simulink model "hr_PID"  (R2024b)
settings: Solver=VariableStepAuto  StartTime=0.0  StopTime=T  RelTol=1e-3
values from neighbouring files (symbols this model uses):
  a = 1    [bifurcation_diagram.m]    (also in equilibria.m; flow.m; flow_analysis.m; linear_analysis.m)
  A = hr_jacobian(x_eq, a, b, d, r, s)    [params.m]
  b = 3    [bifurcation_diagram.m]    (also in equilibria.m; flow.m; flow_analysis.m; linear_analysis.m = linspace(0, 10, 100))
  B = [1; 0; 0]    [params.m]
  c = 1    [bifurcation_diagram.m]    (also in equilibria.m; flow.m; flow_analysis.m; linear_analysis.m)
  C = [1, 0, 0]    [params.m]
  d = 5    [bifurcation_diagram.m]    (also in equilibria.m; flow.m; flow_analysis.m; linear_analysis.m)
  D = 0    [params.m]
  d_filter = 100    [params.m]
  I = linspace(1.2, 3.5, 1000)    [bifurcation_diagram.m]    (also in equilibria.m = 1.309; flow.m = 1.3059; linear_analysis.m = 2; params.m = 1.28)
  Kd = 2.67    [params.m]
  Ki = 49.48    [params.m]
  Kp = 108.97    [params.m]
  r = 0.003    [bifurcation_diagram.m]    (also in equilibria.m; flow.m; flow_analysis.m; linear_analysis.m = 0.001)
  s = 4    [bifurcation_diagram.m]    (also in equilibria.m; flow.m; flow_analysis.m; linear_analysis.m)
  uncertainty = 0    [params.m]    (also in plot_sim_reg.m; plot_sim_reg_disturbance.m; plot_sim_reg_uncertainties.m = 1; plot_sim_track.m)
  x_0 = [0.1; 0.1; 0.1]    [bifurcation_diagram.m]    (also in flow.m = x_0_generic; params.m; plot_sim_track.m = hr_equilibria(a,b,c,d,s,x_r,I); plot_sim_track_disturbance.m = hr_equilibria(a,b,c,d,s,x_r,I))
  x_eq = current_eq(1, j)    [linear_analysis.m]    (also in params.m = eq(1,1); plot_sim_track.m = eq(1,1); plot_sim_track_disturbance.m = eq(1,1); plot_sim_track_uncertainties.m = eq(1,1))
  x_r = -8/5    (= -1.6)    [bifurcation_diagram.m]    (also in equilibria.m; flow.m; flow_analysis.m; linear_analysis.m)
libraries: slpidlib x2
settings Model: Creator=vincip  LastModifiedBy=vincip

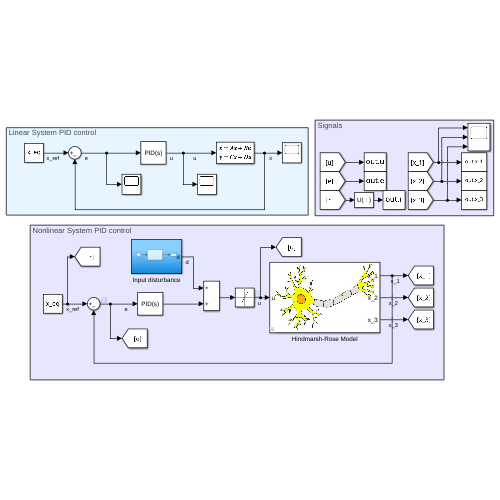
[thumbnail: Simulink's stored preview of the top-level diagram]
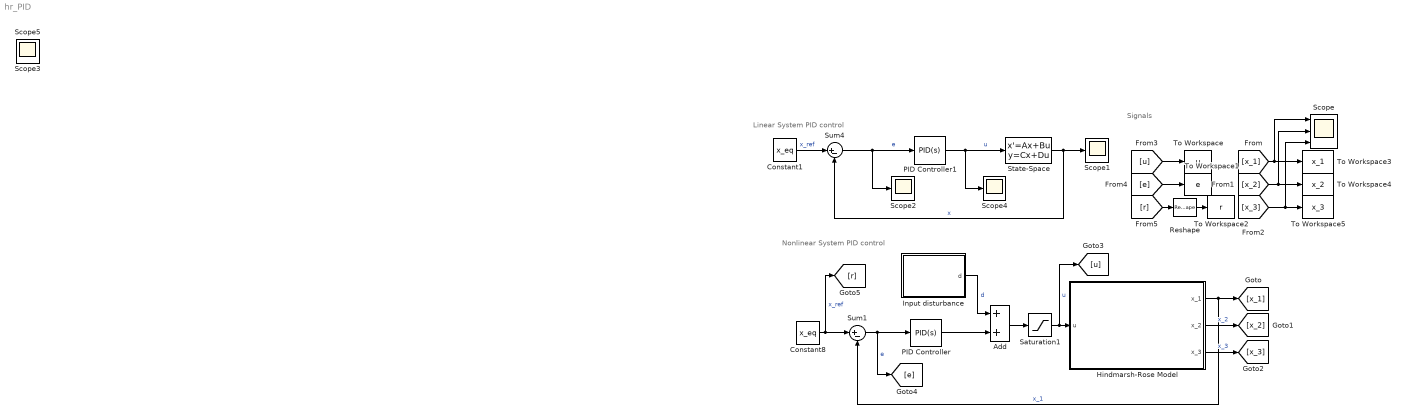
== system hr_PID ==
  note: Signals
  note: Linear System PID control
  note: Nonlinear System PID control
  Add : Sum
  Constant1 : Constant  Value=x_eq
  Constant8 : Constant  Value=x_eq
  Hindmarsh-Rose Model : Subsystem  mask{a=a, b=b, c=c, d=d, r=r, s=s, x_r=x_r, I=I, x_0=x_0, uncertainty=uncertainty}
      mask DialogControl DescTextVar Prompt: Hindmarsh-Rose Neuronal Model with an external input u
      mask Display:
      | image('figures/neuron.jpg');
      | port_label('input', 1, 'u');
      | port_label('output', 1, 'x_1');
      | port_label('output', 2, 'x_2');
      | port_label('output', 3, 'x_3');
  Input disturbance : Subsystem
  PID Controller : slpidlib/PID Controller  Controller=PID  Form=Parallel  TimeDomain=Continuous-time  UseExternalTs=off  SampleTime=-1  IntegratorMethod=Forward Euler  FilterMethod=Forward Euler  ControllerParametersSource=internal  P=Kp  I=Ki  UseKiTs=off  D=Kd  UseExternalDerivativeSource=off  N=d_filter  UseFilter=on  TunerSelectOption=Transfer Function Based (PID Tuner App)  InitialConditionSource=internal  InitialConditionForIntegrator=0  InitialConditionForFilter=0  DifferentiatorICPrevScaledInput=0  ExternalReset=none  TrackingMode=off  Kt=1  LimitOutput=off  SatLimitsSource=internal  UpperSaturationLimit=inf  LowerSaturationLimit=-inf  LinearizeAsGain=on  AntiWindupMode=none  Kb=1  LimitIntegrator=off  UpperIntegratorSaturationLimit=inf  LowerIntegratorSaturationLimit=-inf  POutMin=[]  POutMax=[]  IOutMin=[]  IOutMax=[]  DOutMin=[]  DOutMax=[]  NOutMin=[]  NOutMax=[]  SumOutMin=[]  SumOutMax=[]  SaturationOutMin=[]  SaturationOutMax=[]  PParamMin=[]  PParamMax=[]  IParamMin=[]  IParamMax=[]  DParamMin=[]  DParamMax=[]  NParamMin=[]  NParamMax=[]  KbParamMin=[]  KbParamMax=[]  KtParamMin=[]  KtParamMax=[]  KbOutMin=[]  KbOutMax=[]  KtOutMin=[]  KtOutMax=[]  IntegratorOutMin=[]  IntegratorOutMax=[]  FilterOutMin=[]  FilterOutMax=[]  SumI1OutMin=[]  SumI1OutMax=[]  SumI2OutMin=[]  SumI2OutMax=[]  SumI3OutMin=[]  SumI3OutMax=[]  SumI4OutMin=[]  SumI4OutMax=[]  SumDOutMin=[]  SumDOutMax=[]  DifferentiatorOutMin=[]  DifferentiatorOutMax=[]  FilterDiffOutCoefMin=[]  FilterDiffOutCoefMax=[]  ReciprocalOutMin=[]  ReciprocalOutMax=[]  SumDenOutMin=[]  SumDenOutMax=[]  SumNumOutMin=[]  SumNumOutMax=[]  DivideOutMin=[]  DivideOutMax=[]  UdiffTsProdOutMin=[]  UdiffTsProdOutMax=[]  NTsProdOutMin=[]  NTsProdOutMax=[]  UintegralTsProdOutMin=[]  UintegralTsProdOutMax=[]  UngainTsProdOutMin=[]  UngainTsProdOutMax=[]  ClampingZeroOutDataTypeStr=Inherit: Inherit via back propagation  ClampingZeroOutMin=[]  ClampingZeroOutMax=[]  FilterDenConstantOutDataTypeStr=Inherit: Inherit via back propagation  FilterDenConstantOutMin=[]  FilterDenConstantOutMax=[]  PCopyOutDataTypeStr=Inherit: Inherit via back propagation  PCopyOutMin=[]  PCopyOutMax=[]  NCopyOutDataTypeStr=Inherit: Inherit via back propagation  NCopyOutMin=[]  NCopyOutMax=[]  IntegratorContinuousStateAttributes=''  IntegratorStateMustResolveToSignalObject=off  IntegratorRTWStateStorageClass=Auto  FilterContinuousStateAttributes=''  FilterStateMustResolveToSignalObject=off  FilterRTWStateStorageClass=Auto  ParallelPVariant=InternalParameters  IdealPVariant=Disabled  IVariant=InternalParameters  DVariant=InternalParameters  IntegratorVariant=Continuous  SatVariant=Disabled  AWVariant=Passthrough  PCopyVariant=Disabled  TRVariant=Disabled  FdbkBlocksVariant=Forward  IdealPFdbkVariant=Disabled  SatFdbkVariant=Disabled  DerivativeFilterVariant=ContFilter  NVariant=InternalParameters  NCopyVariant=Disabled  FilterICVariant=InternalICsFilter  IntegratorICVariant=InternalICs  ExternalResetVariant=Disabled  TRSumVariant=Passthrough  SumFdbkVariant=Disabled  SumVariant=Sum_PID  TsampFilterVariant=InternalTs  TsampNgainVariant=Passthrough  TsampIntegralVariant=Disabled_SignalSpec  ExternalSaturationOutDataTypeStr=Inherit: Same as second input  DerivativeSourceVariant=ErrorSignal  PreIntVariant=InternalPreInt
  PID Controller1 : slpidlib/PID Controller  Controller=PID  Form=Parallel  TimeDomain=Continuous-time  UseExternalTs=off  SampleTime=-1  IntegratorMethod=Forward Euler  FilterMethod=Forward Euler  ControllerParametersSource=internal  P=Kp  I=Ki  UseKiTs=off  D=Kd  UseExternalDerivativeSource=off  N=d_filter  UseFilter=on  TunerSelectOption=Transfer Function Based (PID Tuner App)  InitialConditionSource=internal  InitialConditionForIntegrator=0  InitialConditionForFilter=0  DifferentiatorICPrevScaledInput=0  ExternalReset=none  TrackingMode=off  Kt=1  LimitOutput=off  SatLimitsSource=internal  UpperSaturationLimit=inf  LowerSaturationLimit=-inf  LinearizeAsGain=on  AntiWindupMode=none  Kb=1  LimitIntegrator=off  UpperIntegratorSaturationLimit=inf  LowerIntegratorSaturationLimit=-inf  POutMin=[]  POutMax=[]  IOutMin=[]  IOutMax=[]  DOutMin=[]  DOutMax=[]  NOutMin=[]  NOutMax=[]  SumOutMin=[]  SumOutMax=[]  SaturationOutMin=[]  SaturationOutMax=[]  PParamMin=[]  PParamMax=[]  IParamMin=[]  IParamMax=[]  DParamMin=[]  DParamMax=[]  NParamMin=[]  NParamMax=[]  KbParamMin=[]  KbParamMax=[]  KtParamMin=[]  KtParamMax=[]  KbOutMin=[]  KbOutMax=[]  KtOutMin=[]  KtOutMax=[]  IntegratorOutMin=[]  IntegratorOutMax=[]  FilterOutMin=[]  FilterOutMax=[]  SumI1OutMin=[]  SumI1OutMax=[]  SumI2OutMin=[]  SumI2OutMax=[]  SumI3OutMin=[]  SumI3OutMax=[]  SumI4OutMin=[]  SumI4OutMax=[]  SumDOutMin=[]  SumDOutMax=[]  DifferentiatorOutMin=[]  DifferentiatorOutMax=[]  FilterDiffOutCoefMin=[]  FilterDiffOutCoefMax=[]  ReciprocalOutMin=[]  ReciprocalOutMax=[]  SumDenOutMin=[]  SumDenOutMax=[]  SumNumOutMin=[]  SumNumOutMax=[]  DivideOutMin=[]  DivideOutMax=[]  UdiffTsProdOutMin=[]  UdiffTsProdOutMax=[]  NTsProdOutMin=[]  NTsProdOutMax=[]  UintegralTsProdOutMin=[]  UintegralTsProdOutMax=[]  UngainTsProdOutMin=[]  UngainTsProdOutMax=[]  ClampingZeroOutDataTypeStr=Inherit: Inherit via back propagation  ClampingZeroOutMin=[]  ClampingZeroOutMax=[]  FilterDenConstantOutDataTypeStr=Inherit: Inherit via back propagation  FilterDenConstantOutMin=[]  FilterDenConstantOutMax=[]  PCopyOutDataTypeStr=Inherit: Inherit via back propagation  PCopyOutMin=[]  PCopyOutMax=[]  NCopyOutDataTypeStr=Inherit: Inherit via back propagation  NCopyOutMin=[]  NCopyOutMax=[]  IntegratorContinuousStateAttributes=''  IntegratorStateMustResolveToSignalObject=off  IntegratorRTWStateStorageClass=Auto  FilterContinuousStateAttributes=''  FilterStateMustResolveToSignalObject=off  FilterRTWStateStorageClass=Auto  ParallelPVariant=InternalParameters  IdealPVariant=Disabled  IVariant=InternalParameters  DVariant=InternalParameters  IntegratorVariant=Continuous  SatVariant=Disabled  AWVariant=Passthrough  PCopyVariant=Disabled  TRVariant=Disabled  FdbkBlocksVariant=Forward  IdealPFdbkVariant=Disabled  SatFdbkVariant=Disabled  DerivativeFilterVariant=ContFilter  NVariant=InternalParameters  NCopyVariant=Disabled  FilterICVariant=InternalICsFilter  IntegratorICVariant=InternalICs  ExternalResetVariant=Disabled  TRSumVariant=Passthrough  SumFdbkVariant=Disabled  SumVariant=Sum_PID  TsampFilterVariant=InternalTs  TsampNgainVariant=Passthrough  TsampIntegralVariant=Disabled_SignalSpec  ExternalSaturationOutDataTypeStr=Inherit: Same as second input  DerivativeSourceVariant=ErrorSignal  PreIntVariant=InternalPreInt
  Reshape : Reshape
  Saturation1 : Saturate  UpperLimit=10  LowerLimit=-10  LinearizeAsGain=off  ZeroCross=off
  Scope : Scope  NumInputPorts=3
  Scope{1..5} (5 alike) : Scope
  State-Space : StateSpace  A=A  B=B  C=C  D=D  InitialCondition=x_0
  Sum1 : Sum  Inputs=|+-
  Sum4 : Sum  Inputs=|+-
  To Workspace : ToWorkspace  VariableName=u  SaveFormat=Timeseries  SampleTime=-1
  To Workspace1 : ToWorkspace  VariableName=e  SaveFormat=Timeseries  SampleTime=-1
  To Workspace2 : ToWorkspace  VariableName=r  SaveFormat=Timeseries  SampleTime=-1
  To Workspace3 : ToWorkspace  VariableName=x_1  SaveFormat=Timeseries  SampleTime=-1
  To Workspace4 : ToWorkspace  VariableName=x_2  SaveFormat=Timeseries  SampleTime=-1
  To Workspace5 : ToWorkspace  VariableName=x_3  SaveFormat=Timeseries  SampleTime=-1
  wires:
  Constant8/1 -> [r], Sum1/1  "x_ref"
  PID Controller/1 -> Add/2
  Add/1 -> Saturation1/1
  Sum1/1 -> [e], PID Controller/1  "e"
  PID Controller1/1 -> State-Space/1, Scope4/1  "u"
  Sum4/1 -> Scope2/1, PID Controller1/1  "e"
  Constant1/1 -> Sum4/1  "x_ref"
  State-Space/1 -> Scope1/1, Sum4/2  "x"
  Input disturbance/1(d) -> Add/1  "d"
  Saturation1/1 -> [u], Hindmarsh-Rose Model/1(u)  "u"
  Hindmarsh-Rose Model/2(x_2) -> [x_2]  "x_2"
  Hindmarsh-Rose Model/3(x_3) -> [x_3]  "x_3"
  Hindmarsh-Rose Model/1(x_1) -> Sum1/2, [x_1]  "x_1"
  [x_1] -> To Workspace3/1, Scope/1
  [x_2] -> To Workspace4/1, Scope/2
  [x_3] -> To Workspace5/1, Scope/3
  [u] -> To Workspace/1
  [e] -> To Workspace1/1
  [r] -> Reshape/1
  Reshape/1 -> To Workspace2/1

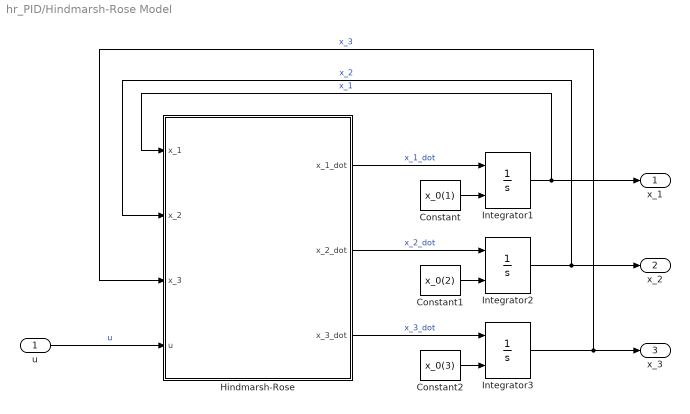
== system hr_PID/Hindmarsh-Rose Model ==
  u : Inport
  Constant : Constant  Value=x_0(1)
  Constant1 : Constant  Value=x_0(2)
  Constant2 : Constant  Value=x_0(3)
  Hindmarsh-Rose : MATLAB Function  TreatAsAtomicUnit=on
  Integrator1 : Integrator  InitialConditionSource=external  InitialCondition=x_0
  Integrator2 : Integrator  InitialConditionSource=external  InitialCondition=x_0
  Integrator3 : Integrator  InitialConditionSource=external  InitialCondition=x_0
  x_1 : Outport
  x_2 : Outport  Port=2
  x_3 : Outport  Port=3
  wires:
  Hindmarsh-Rose/2(x_2_dot) -> Integrator2/1  "x_2_dot"
  Integrator1/1 -> Hindmarsh-Rose/1(x_1), x_1/1  "x_1"
  Hindmarsh-Rose/3(x_3_dot) -> Integrator3/1  "x_3_dot"
  Integrator3/1 -> x_3/1, Hindmarsh-Rose/3(x_3)  "x_3"
  u/1 -> Hindmarsh-Rose/4(u)  "u"
  Hindmarsh-Rose/1(x_1_dot) -> Integrator1/1  "x_1_dot"
  Integrator2/1 -> Hindmarsh-Rose/2(x_2), x_2/1  "x_2"
  Constant/1 -> Integrator1/2
  Constant1/1 -> Integrator2/2
  Constant2/1 -> Integrator3/2

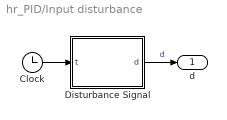
== system hr_PID/Input disturbance ==
  Clock : Clock
  Disturbance Signal : MATLAB Function  TreatAsAtomicUnit=on
  d : Outport
  wires:
  Clock/1 -> Disturbance Signal/1(t)
  Disturbance Signal/1(d) -> d/1  "d"

== matlab function hr_PID/Hindmarsh-Rose Model/Hindmarsh-Rose ==
  data: x_1 input; x_2 input; x_3 input; u input; x_1_dot output; x_2_dot output; x_3_dot output; a parameter; b parameter; c parameter; d parameter; s parameter; r parameter; x_r parameter; I parameter; uncertainty parameter
function [x_1_dot, x_2_dot, x_3_dot]  = hrindmarsh_rose_model(x_1, x_2, x_3, ...
    u, a, b, c, d, s, r, x_r, I, uncertainty)
    % potential uncertainty
    delta = 0.1;
    if uncertainty == 1
        a_real = a*(1 + delta);
        b_real = b*(1 + delta);
        c_real = c*(1 + delta);
        d_real = d*(1 + delta);
    else
        a_real = a;
        b_real = b;
        c_real = c;
        d_real = d;
    end
    % Neuronal model - Hindmarsh Rose
    x_1_dot = x_2 - a_real*x_1^3 + b_real*x_1^2 - x_3 + I + u;
    x_2_dot = c_real - d_real*x_1^2 - x_2;
    x_3_dot = r*(s*(x_1 - x_r) - x_3);

== matlab function hr_PID/Input disturbance/Disturbance Signal ==
  data: d output; t input; choice parameter
function d = disturbance(t, choice)
% Select input disturbance based on the choice parameter
ampl = 0.5;
w = 2*pi * 0.2;
if choice == 1
    d = ampl * sin(w * t);
elseif choice == 2
    if t >= 1.0
        d = 1.0;
    else 
        d = 0.0;
    end
else
    d = 0;
end
